simulink subsystem "Cuk_Inverter"  (R2024a)
settings: Solver=VariableStepAuto  StartTime=0.0  StopTime=10.0  RelTol=1e-3
model mask{Vin=30, Vout_Expect=40, Fsw=100e3, detaIL1=0.1, detaIL2=0.1, detaUC1=0.1, detaUC2=0.1}
  mask prompts: Fsw "Switch Frequency"; detaIL1 "电感纹波"; detaIL2 "电感纹波"; detaUC1 "电压纹波"; detaUC2 "电压纹波"
libraries: spsSeriesRLCBranchLib x4, spsDiodeLib x1, spsMosfetLib x1
settings Model: Creator=ZE  LastModifiedBy=ZE

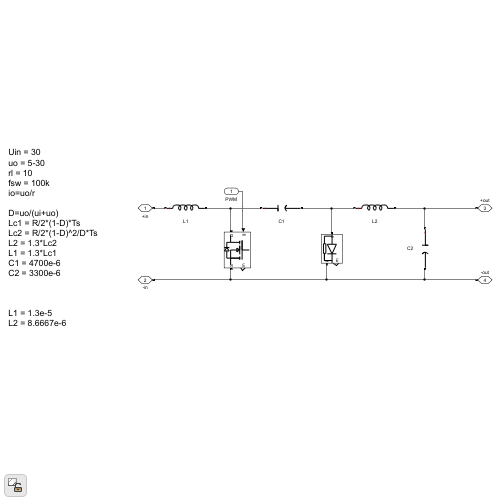
[thumbnail: Simulink's stored preview of the top-level diagram]
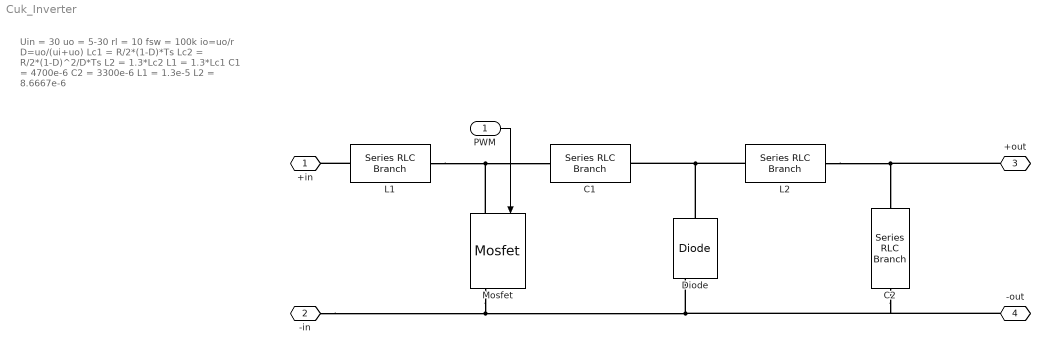
== system Cuk_Inverter ==
  note: Uin = 30
      | uo = 5-30
      | rl = 10
      | fsw = 100k
      | io=uo/r
      |
      | D=uo/(ui+uo)
      | Lc1 = R/2*(1-D)*Ts
      | Lc2 = R/2*(1-D)^2/D*Ts
      | L2 = 1.3*Lc2
      | L1 = 1.3*Lc1
      | C1 = 4700e-6
      | C2 = 3300e-6
      |
      | L1 = 1.3e-5
      | L2 = 8.6667e-6
  PWM : Inport
  C1 : spsSeriesRLCBranchLib/Series RLC Branch  LConnTagsString=__new0  RConnTagsString=__new0  BranchType=C  Resistance=1  Inductance=1e-3  SetiL0=off  InitialCurrent=0  Capacitance=0.0047  Setx0=off  InitialVoltage=0  Measurements=None
  C2 : spsSeriesRLCBranchLib/Series RLC Branch  LConnTagsString=__new0  RConnTagsString=__new0  BranchType=C  Resistance=1  Inductance=1e-3  SetiL0=off  InitialCurrent=0  Capacitance=0.0033  Setx0=off  InitialVoltage=0  Measurements=None
  Diode : spsDiodeLib/Diode  Ron=0.001  Lon=0  Vf=0.8  IC=0  UseSnubber=0  Rs=500  Cs=250e-9  Measurements=on
  L1 : spsSeriesRLCBranchLib/Series RLC Branch  LConnTagsString=__new0  RConnTagsString=__new0  BranchType=L  Resistance=1  Inductance=1.3e-5  SetiL0=off  InitialCurrent=0  Capacitance=1e-6  Setx0=off  InitialVoltage=0  Measurements=None
  L2 : spsSeriesRLCBranchLib/Series RLC Branch  LConnTagsString=__new0  RConnTagsString=__new0  BranchType=L  Resistance=1  Inductance=8.6667e-6  SetiL0=off  InitialCurrent=0  Capacitance=1e-6  Setx0=off  InitialVoltage=0  Measurements=None
  Mosfet : spsMosfetLib/Mosfet  Ron=0.1  Lon=0  Rd=0.01  Vfd=0  IC=0  Rs=1e5  Cs=inf  Measurements=on
  +in : PMIOPort  Side=Left
  -in : PMIOPort  Port=2  Side=Left
  +out : PMIOPort  Port=3  Side=Right
  -out : PMIOPort  Port=4  Side=Right
  wires:
  PWM/1 -> Mosfet/1
  connections:
  L2/RConn1 -- C2/LConn1 -- +out/RConn1
  L2/LConn1 -- C1/RConn1 -- Diode/LConn1
  L1/RConn1 -- C1/LConn1 -- Mosfet/LConn1
  Mosfet/RConn1 -- Diode/RConn1 -- C2/RConn1 -- -out/RConn1 -- -in/RConn1
  L1/LConn1 -- +in/RConn1
